simulink subsystem "ControlLedsFinal"  (R2021b)
settings: Solver=VariableStepAuto  StartTime=0.0  StopTime=10.0  RelTol=1e-3
libraries: arduinolib x3, simulink x1, commutil2 x1
settings Model: Creator=yo  LastModifiedBy=ferna

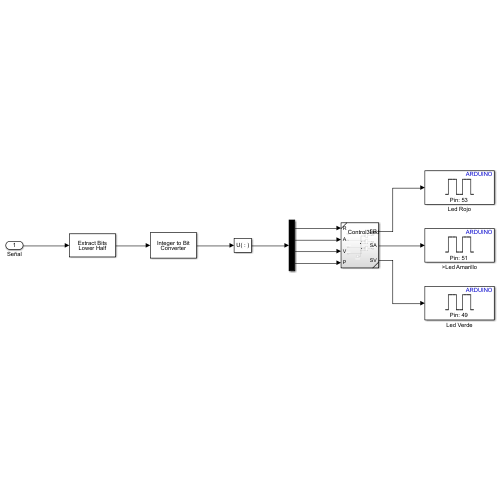
[thumbnail: Simulink's stored preview of the top-level diagram]
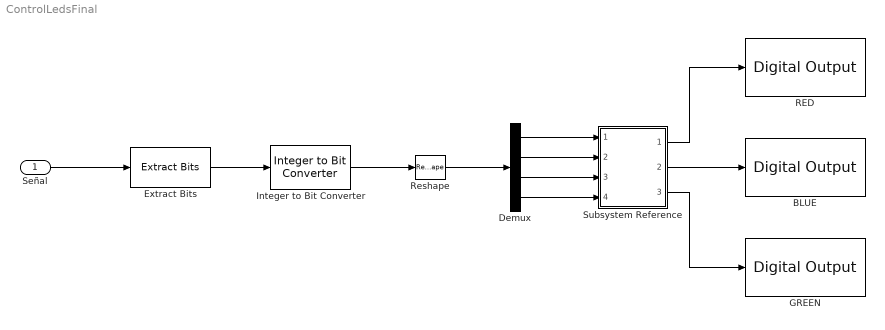
== system ControlLedsFinal ==
  Señal : Inport
  BLUE : arduinolib/Digital Output  pinNumber=53  Direction=output  blockPlatform=arduino
  Demux : Demux
  Extract Bits : simulink/Logic and Bit Operations/Extract Bits  bitsToExtract=Lower half  numBits=8  bitIdxRange=[0 3]  outScalingMode=Preserve fixed-point scaling
  GREEN : arduinolib/Digital Output  pinNumber=51  Direction=output  blockPlatform=arduino
  Integer to Bit Converter : commutil2/Integer to Bit Converter  nbits=4  signedInputValues=Unsigned  bitOrder=MSB first  outDtype=Inherit via internal rule
  RED : arduinolib/Digital Output  pinNumber=49  Direction=output  blockPlatform=arduino
  Reshape : Reshape
  Subsystem Reference : Subsystem  ReferencedSubsystem=Control3Leds
  wires:
  Demux/3 -> Subsystem Reference/3
  Demux/2 -> Subsystem Reference/2
  Subsystem Reference/2 -> BLUE/1
  Demux/4 -> Subsystem Reference/4
  Extract Bits/1 -> Integer to Bit Converter/1
  Subsystem Reference/3 -> GREEN/1
  Reshape/1 -> Demux/1
  Integer to Bit Converter/1 -> Reshape/1
  Demux/1 -> Subsystem Reference/1
  Señal/1 -> Extract Bits/1
  Subsystem Reference/1 -> RED/1
